simulink model "QuadrotorSimulink_w_memory_cex"  (R2020a)
settings: Solver=FixedStepAuto  StartTime=0.0  StopTime=options.T_train  FixedStep=options.dt  RelTol=1e-6
undefined symbols (not defined in the file or in its folder): options, Quad
libraries: neural x179, simulink x2
(part 5 of 10)

== system QuadrotorSimulink_w_memory_cex/NN/Layer 2/Delays 1 ==
  "p{2}" : Inport  PortDimensions=50
      mask Display: e = 0.06;c1 = [120 230 180]/255;c2 = ([120 230 180]+0)/(256+128);c3 = ([120 230 180]+128)/(256+128);patch([0 1 1 0],[0 0 1 1],c1);patch([0 1 1 1-e 1-e 0+e],[0 0 1 1-e 0+e 0+e],c2);patch([0 0 1 1-e 0+e 0+e],[0 1 1 1-e 1-e 0+e],c3);plot([0 1 1 0 0],[0 0 1 1 0]);
  mux : Mux  Inputs=1
      mask Display: e = 0.06;c1 = [120 150 230]/255;c2 = ([120 150 230]+0)/383;c3 = ([120 150 230]+128)/383;patch([0 1 1 0],[0 0 1 1],c1);patch([0 1 1 1-e 1-e 0+e],[0 0 1 1-e 0+e 0+e],c2);patch([0 0 1 1-e 0+e 0+e],[0 1 1 1-e 1-e 0+e],c3);plot([0 1 1 0 0],[0 0 1 1 0]);disp('Mux')
  "pd{2,1}" : Outport
      mask Display: e = 0.06;c1 = [120 230 180]/255;c2 = ([120 230 180]+0)/(256+128);c3 = ([120 230 180]+128)/(256+128);patch([0 1 1 0],[0 0 1 1],c1);patch([0 1 1 1-e 1-e 0+e],[0 0 1 1-e 0+e 0+e],c2);patch([0 0 1 1-e 0+e 0+e],[0 1 1 1-e 1-e 0+e],c3);plot([0 1 1 0 0],[0 0 1 1 0]);
  wires:
  "p{2}"/1 -> mux/1
  mux/1 -> "pd{2,1}"/1

== system QuadrotorSimulink_w_memory_cex/NN/Layer 2/LW{2,1} ==
  "ad{2,1}" : Inport  PortDimensions=50
      mask Display: e = 0.06;c1 = [120 230 180]/255;c2 = ([120 230 180]+0)/(256+128);c3 = ([120 230 180]+128)/(256+128);patch([0 1 1 0],[0 0 1 1],c1);patch([0 1 1 1-e 1-e 0+e],[0 0 1 1-e 0+e 0+e],c2);patch([0 0 1 1-e 0+e 0+e],[0 1 1 1-e 1-e 0+e],c3);plot([0 1 1 0 0],[0 0 1 1 0]);
  "IW{2,1}(1,:)'" : Constant  Value=[0.279690236721947871334492674577631987631320953369140625;0.2177538111736299075715805884101428091526031494140625;-0.05749136422813690139310693894003634341061115264892578125;-0.82599074193307819857778895311639644205570220947265625;-0.048836686517867093637601527689184877090156078338623046875;-0.1087265384554891578527957562982919625937938690185546875;-0.88600682883338510720250269514508545398712158203125;0.008264634763566834629866519890128984116017818450927734375;2.112115039147600459301656883326359093189239501953125;-0.1706783234922826519852634419294190593063831329345703125;-2.538082397267302336985039801220409572124481201171875;-0.71040606190064903291414566410821862518787384033203125;-1.971265049043579242749046898097731173038482666015625;2.7124696631005775770972832106053829193115234375;-0.20875006868320433728314355903421528637409210205078125;-0.476172145987987127657703467775718308985233306884765625;-1.6561068348180285614290596640785224735736846923828125;0.273719643821595581822947451655636541545391082763671875;0.1539877606696956335863291087662219069898128509521484375;0.09163426395482125730307387811990338377654552459716796875;-0.60014325523041378573907422833144664764404296875;-2.717758758867210300280703449971042573451995849609375;-2.772479731221027865473161000409163534641265869140625;0.307198293656782250860004523929092101752758026123046875;0.211829192148631662018232191257993690669536590576171875;-0.61681588760544781013805959446472115814685821533203125;0.195041689330810896763068740256130695343017578125;0.06706954206715602662125519373148563317954540252685546875;-0.07494671086691785666378251562491641379892826080322265625;1.8960268372474338161026707894052378833293914794921875;-1.319010769993005371958361138240434229373931884765625;-4.61269853580427113826090135262347757816314697265625;1.4754426327383616257549192596343345940113067626953125;-0.75849083803097017142391678135027177631855010986328125;0.14406042025683818419423687373637221753597259521484375;1.9329867207918010052480894955806434154510498046875;3.41057221623705775215285029844380915164947509765625;0.3135240703596695599486565697588957846164703369140625;2.1135026100098333046162224491126835346221923828125;1.2970714038750263963351017082459293305873870849609375;3.214326785540090103410193478339351713657379150390625;1.3362962255985781911959975332138128578662872314453125;0.146731693279233521565174669376574456691741943359375;0.3330503193597691424798767911852337419986724853515625;-0.66352017059547774291416999403736554086208343505859375;-0.2412462434265259247911927786844898946583271026611328125;0.11662064695715369799788874161095009185373783111572265625;-0.88981112191568223490634181871428154408931732177734375;1.1406275449783009889870299957692623138427734375;0.04197529870444034749699113717724685557186603546142578125]
      mask Display: e = 0.06;c1 = [120 150 230]/255;c2 = ([120 150 230]+0)/383;c3 = ([120 150 230]+128)/383;patch([0 1 1 0],[0 0 1 1],c1);patch([0 1 1 1-e 1-e 0+e],[0 0 1 1-e 0+e 0+e],c2);patch([0 0 1 1-e 0+e 0+e],[0 1 1 1-e 1-e 0+e],c3);plot([0 1 1 0 0],[0 0 1 1 0]);disp('weights');
  "IW{2,1}(2,:)'" : Constant  Value=[-0.1552708258403756313992261084422352723777294158935546875;-0.375819834139433484043735234081395901739597320556640625;-0.005011030686745109215263216384528277558274567127227783203125;0.356927115853283627444625381031073629856109619140625;-0.310289415245989796954262374129029922187328338623046875;0.307477983563482271112121679834672249853610992431640625;2.424113781658061572699125463259406387805938720703125;-0.77393457089228590017881970197777263820171356201171875;0.521993923742927190545515259145759046077728271484375;-0.1944574914692172862284991197157069109380245208740234375;-0.4012363429594547614698285542544908821582794189453125;0.315113917795899312057628094407846219837665557861328125;-1.273241940356574009030055094626732170581817626953125;2.743669051586928642194607164128683507442474365234375;-0.0966473291433087577928517930558882653713226318359375;0.053270004543143643915836804580976604484021663665771484375;-1.16597425841194990425719879567623138427734375;0.258584706191077484671581032671383582055568695068359375;0.54299192984982436183116760730626992881298065185546875;0.0245356508001520583206467307491038809530436992645263671875;1.567586920662038973972585154115222394466400146484375;2.372265239968957217797651537694036960601806640625;2.03356924194495025659534803708083927631378173828125;0.0288152173723420050588384100365146878175437450408935546875;-0.31763376195907888632774529469315893948078155517578125;-0.0980309890113009174683611490763723850250244140625;0.432665787132838153272729186937795020639896392822265625;-0.034388383686032551744826690764966770075261592864990234375;-0.02981958460602428251373652301481342874467372894287109375;0.3690270055964119944036383458296768367290496826171875;-1.54508949896811742519275867380201816558837890625;-0.1028872647031311704513001359373447485268115997314453125;-0.345866568600938728561544621697976253926753997802734375;0.02182718731870815498385951514137559570372104644775390625;0.1995526466919978758607356894572149030864238739013671875;2.080251365431149412899003436905331909656524658203125;1.5525275121063064620585691955056972801685333251953125;0.065141767169451025853987857772153802216053009033203125;-0.36549041295080264557526561475242488086223602294921875;0.2440044620822674759086368112548370845615863800048828125;-1.8752978872370056340201927014277316629886627197265625;-1.16282625407332940170590518391691148281097412109375;0.2336982340092603471770615897185052745044231414794921875;0.499794504720247056983595257406705059111118316650390625;0.273739985432975230228436203105957247316837310791015625;-0.0762427898702588702217752825163188390433788299560546875;-0.8515688371054934702186756112496368587017059326171875;0.96090733448069698408033900705049745738506317138671875;-0.344915244349439820137348533535259775817394256591796875;-1.292928046065546343612595592276193201541900634765625]
      mask Display: e = 0.06;c1 = [120 150 230]/255;c2 = ([120 150 230]+0)/383;c3 = ([120 150 230]+128)/383;patch([0 1 1 0],[0 0 1 1],c1);patch([0 1 1 1-e 1-e 0+e],[0 0 1 1-e 0+e 0+e],c2);patch([0 0 1 1-e 0+e 0+e],[0 1 1 1-e 1-e 0+e],c3);plot([0 1 1 0 0],[0 0 1 1 0]);disp('weights');
  Mux : Mux  Inputs=2
      mask Display: e = 0.06;c1 = [120 150 230]/255;c2 = ([120 150 230]+0)/383;c3 = ([120 150 230]+128)/383;patch([0 1 1 0],[0 0 1 1],c1);patch([0 1 1 1-e 1-e 0+e],[0 0 1 1-e 0+e 0+e],c2);patch([0 0 1 1-e 0+e 0+e],[0 1 1 1-e 1-e 0+e],c3);plot([0 1 1 0 0],[0 0 1 1 0]);disp('Mux');
  dotprod1 : neural/Weight Functions/dotprod
  dotprod2 : neural/Weight Functions/dotprod
  "lz{2,1}" : Outport
      mask Display: e = 0.06;c1 = [120 230 180]/255;c2 = ([120 230 180]+0)/(256+128);c3 = ([120 230 180]+128)/(256+128);patch([0 1 1 0],[0 0 1 1],c1);patch([0 1 1 1-e 1-e 0+e],[0 0 1 1-e 0+e 0+e],c2);patch([0 0 1 1-e 0+e 0+e],[0 1 1 1-e 1-e 0+e],c3);plot([0 1 1 0 0],[0 0 1 1 0]);
  wires:
  "IW{2,1}(1,:)'"/1 -> dotprod1/1
  "ad{2,1}"/1 -> dotprod1/2, dotprod2/2
  dotprod1/1 -> Mux/1
  "IW{2,1}(2,:)'"/1 -> dotprod2/1
  dotprod2/1 -> Mux/2
  Mux/1 -> "lz{2,1}"/1

== system QuadrotorSimulink_w_memory_cex/NN_cex_1/Layer 1/Delays 1 ==
  "p{1}" : Inport  PortDimensions=15
      mask Display: e = 0.06;c1 = [120 230 180]/255;c2 = ([120 230 180]+0)/(256+128);c3 = ([120 230 180]+128)/(256+128);patch([0 1 1 0],[0 0 1 1],c1);patch([0 1 1 1-e 1-e 0+e],[0 0 1 1-e 0+e 0+e],c2);patch([0 0 1 1-e 0+e 0+e],[0 1 1 1-e 1-e 0+e],c3);plot([0 1 1 0 0],[0 0 1 1 0]);
  mux : Mux  Inputs=1
      mask Display: e = 0.06;c1 = [120 150 230]/255;c2 = ([120 150 230]+0)/383;c3 = ([120 150 230]+128)/383;patch([0 1 1 0],[0 0 1 1],c1);patch([0 1 1 1-e 1-e 0+e],[0 0 1 1-e 0+e 0+e],c2);patch([0 0 1 1-e 0+e 0+e],[0 1 1 1-e 1-e 0+e],c3);plot([0 1 1 0 0],[0 0 1 1 0]);disp('Mux')
  "pd{1,1}" : Outport
      mask Display: e = 0.06;c1 = [120 230 180]/255;c2 = ([120 230 180]+0)/(256+128);c3 = ([120 230 180]+128)/(256+128);patch([0 1 1 0],[0 0 1 1],c1);patch([0 1 1 1-e 1-e 0+e],[0 0 1 1-e 0+e 0+e],c2);patch([0 0 1 1-e 0+e 0+e],[0 1 1 1-e 1-e 0+e],c3);plot([0 1 1 0 0],[0 0 1 1 0]);
  wires:
  "p{1}"/1 -> mux/1
  mux/1 -> "pd{1,1}"/1
